simulink model "s0501_rollest_rideheight"  (R2021a)
settings: Solver=FixedStepAuto  StartTime=0.0  StopTime=10.0  FixedStep=0.001  RelTol=1e-3
libraries: CarMaker4SL x27, dspfdesign x1
settings Model: Creator=jason  LastModifiedBy=jason
settings ModelReferenceCC: ModelReferenceNumInstancesAllowed=Single

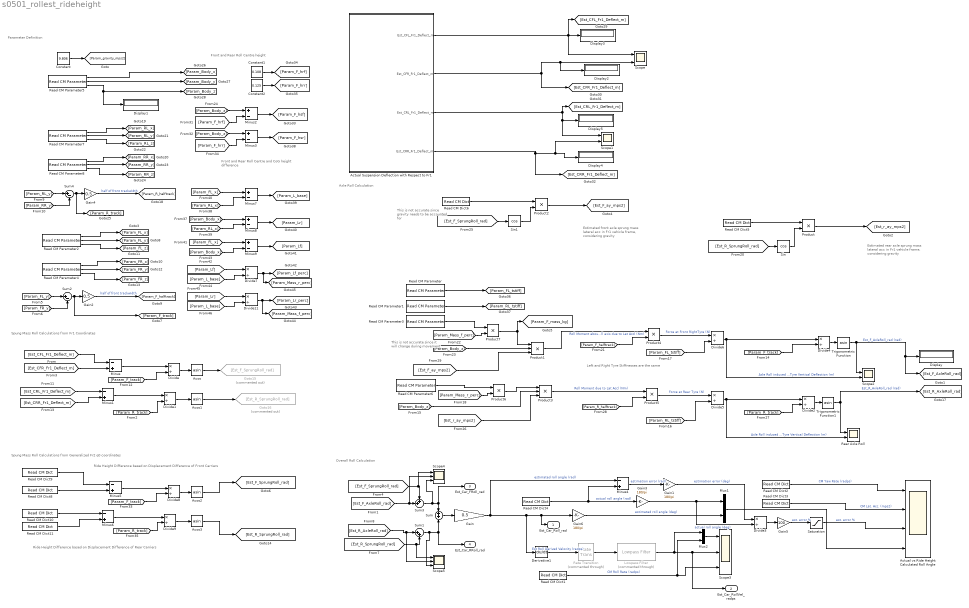
== system s0501_rollest_rideheight ==
  note: Ride Height Difference based on Displacement Difference of Rear Carriers
  note: Ride Height Difference based on Displacement Difference of Front Carriers
  note: Front and Rear Roll Centre height
  note: Overall Roll Calculation
  note: Parameter Definition
  note: Axle Roll Calculation
  note: Left and Right Tyre Stiffnesses are the same
  note: Spung Mass Roll Calculations from Fr1 Coordinates
  note: Estimated front axle sprung mass lateral acc in Fr1 vehicle frame, considering gravity
  note: Spung Mass Roll Calculations from Generalized Fr2 q0 coordinates
  note: This is not accurate since it will change during movement
  note: This is not accurate since gravity needs to be accounted for
  note: Estimated rear axle sprung mass lateral acc in Fr1 vehicle frame, considering gravity
  note: Front and Rear Roll Centre and CoG height difference
  Acos{,1..3} (4 alike) : Trigonometry  Operator=asin
  Actual Suspension Deflection with Respect to Fr1 : Subsystem
  Actual vs Ride Height Calculated Roll Angle : Scope  NumInputPorts=4
  Constant : Constant  Value=9.806
  Constant1 : Constant  Value=0.108
  Constant2 : Constant  Value=0.125
  Derivative1 : Derivative
  Display{,1..5} (6 alike) : Display
  Divide{,1..9,11} (11 alike) : Product  Inputs=*/
  Gain : Gain  Gain=0.5
  Gain1 : Gain  Gain=180/pi
      settings: AttributesFormatString=Gain = %<Gain>
  Gain2 : Gain  Gain=0.5
  Gain3 : Gain  Gain=180/pi
      settings: AttributesFormatString=Gain = %<Gain>
  Gain4 : Gain  Gain=0.5
  Gain5 : Gain  Gain=100
  Gain6 : Gain  Gain=180/pi
      settings: AttributesFormatString=Gain = %<Gain>
  Goto15 : Goto  Commented=on  GotoTag=Est_F_SprungRoll_rad
  Goto16 : Goto  Commented=on  GotoTag=Est_R_SprungRoll_rad
  Lowpass Filter : dspfdesign/Lowpass Filter  Commented=through  FilterType=FIR  DesignForMinimumOrder=on  FilterOrder=50  PassbandFrequency=1  StopbandFrequency=2000  PassbandRipple=0.1  StopbandAttenuation=180  InheritSampleRate=off  SampleRate=44100  SimulateUsing=Interpreted execution  roundingMode=Floor  coeffsDataTypeStr=fixdt(1,16)
  Minus{,1,4..6} (5 alike) : Sum  Inputs=-+
  Minus{2..3,7..9} (5 alike) : Sum  Inputs=+-
  Mux1 : Mux  Inputs=2
  Mux2 : Mux  Inputs=2
  Product{,2,4..7} (6 alike) : Product
  Product1 : Product  Inputs=3
  Product3 : Product  Inputs=3
  Rate Transition : RateTransition  Commented=through
  Read CM Dict1 : CarMaker4SL/Read CM Dict  xname=Car.RollVel  xsync=off  xstime=Continuous
  Read CM Dict10 : CarMaker4SL/Read CM Dict  xname=Car.CRL.q0  xsync=off  xstime=Continuous
  Read CM Dict11 : CarMaker4SL/Read CM Dict  xname=Car.CRR.q0  xsync=off  xstime=Continuous
  Read CM Dict2 : CarMaker4SL/Read CM Dict  xname=Car.YawRate  xsync=off  xstime=Continuous
  Read CM Dict3 : CarMaker4SL/Read CM Dict  xname=Car.ay  xsync=off  xstime=Continuous
  Read CM Dict4 : CarMaker4SL/Read CM Dict  xname=Car.Roll  xsync=off  xstime=Continuous
  Read CM Dict5 : CarMaker4SL/Read CM Dict  xname=Car.ay  xsync=off  xstime=Continuous
  Read CM Dict6 : CarMaker4SL/Read CM Dict  xname=Car.ay  xsync=off  xstime=Continuous
  Read CM Dict8 : CarMaker4SL/Read CM Dict  xname=Car.CFR.q0  xsync=off  xstime=Continuous
  Read CM Dict9 : CarMaker4SL/Read CM Dict  xname=Car.CFL.q0  xsync=off  xstime=Continuous
  Read CM Parameter : CarMaker4SL/Read CM Parameter  xfile=TireFL  xkey=Radial.Stiffness  xnout=1  xdefaults=0  xmuxed=on  xstime=Continuous
      settings: SourceProductName=CarMaker4SL
  Read CM Parameter1 : CarMaker4SL/Read CM Parameter  xfile=TireRL  xkey=Radial.Stiffness  xnout=1  xdefaults=0  xmuxed=on  xstime=Continuous
      settings: SourceProductName=CarMaker4SL
  Read CM Parameter2 : CarMaker4SL/Read CM Parameter  xfile=Vehicle  xkey=WheelCarrier.fl.pos  xnout=3  xdefaults=eps  xmuxed=off  xstime=Continuous
      settings: SourceProductName=CarMaker4SL
  Read CM Parameter3 : CarMaker4SL/Read CM Parameter  xfile=Vehicle  xkey=Body.mass  xnout=1  xdefaults=eps  xmuxed=off  xstime=Continuous
      settings: SourceProductName=CarMaker4SL
  Read CM Parameter4 : CarMaker4SL/Read CM Parameter  xfile=Vehicle  xkey=WheelCarrier.fr.pos  xnout=3  xdefaults=eps  xmuxed=off  xstime=Continuous
      settings: SourceProductName=CarMaker4SL
  Read CM Parameter5 : CarMaker4SL/Read CM Parameter  xfile=Vehicle  xkey=Body.pos  xnout=3  xdefaults=eps  xmuxed=off  xstime=Continuous
      settings: SourceProductName=CarMaker4SL
  Read CM Parameter6 : CarMaker4SL/Read CM Parameter  xfile=Vehicle  xkey=Body.mass  xnout=1  xdefaults=eps  xmuxed=off  xstime=Continuous
      settings: SourceProductName=CarMaker4SL
  Read CM Parameter7 : CarMaker4SL/Read CM Parameter  xfile=Vehicle  xkey=WheelCarrier.rl.pos  xnout=3  xdefaults=eps  xmuxed=off  xstime=Continuous
      settings: SourceProductName=CarMaker4SL
  Read CM Parameter8 : CarMaker4SL/Read CM Parameter  xfile=Vehicle  xkey=WheelCarrier.rr.pos  xnout=3  xdefaults=eps  xmuxed=off  xstime=Continuous
      settings: SourceProductName=CarMaker4SL
  Rear Axle Roll : Scope  NumInputPorts=2
  Saturation : Saturate  UpperLimit=100  LowerLimit=-100
  Scope{,3..5} (4 alike) : Scope  NumInputPorts=3
  Scope1 : Scope  NumInputPorts=2
  Scope2 : Scope  NumInputPorts=2
  Sin : Trigonometry  Operator=cos
  Sin1 : Trigonometry  Operator=cos
  Sum : Sum  Inputs=+|+
  Sum1 : Sum  Inputs=|++
  Sum2 : Sum  Inputs=|+-
  Sum3 : Sum  Inputs=++|
  Sum4 : Sum  Inputs=|+-
  Trigonometric Function : Trigonometry  Operator=asin
  Trigonometric Function1 : Trigonometry  Operator=asin
  Est_Car_Roll_rad : Outport
  Est_Car_RollVel_radps : Outport  Port=2
  Est_Car_FRoll_rad : Outport  Port=3
  Est_Car_RRoll_rad : Outport  Port=4
  wires:
  [Param_F_track] -> Divide8/2
  [Param_RR_y] -> Sum4/2
  Minus5/1 -> Divide8/1
  Read CM Dict3/1 -> Actual vs Ride Height Calculated Roll Angle/2  "CM Lat. Acc. (mps2)"
  Divide/1 -> Acos/1
  [Est_CRL_Fr1_Deflect_m] -> Minus1/1
  Rate Transition/1 -> Lowpass Filter/1
  Gain1/1 -> Divide3/1  "estimation error (deg)"
  Read CM Parameter3/1 -> Product7/1
  Sin/1 -> Product/2
  Read CM Dict2/1 -> Actual vs Ride Height Calculated Roll Angle/1  "CM Yaw Rate (radps)"
  Acos2/1 -> [Est_F_SprungRoll_rad]
  Acos3/1 -> [Est_R_SprungRoll_rad]
  [Est_F_SprungRoll_rad] -> Sin1/1
  Read CM Parameter4/2 -> [Param_FR_y]
  Gain/1 -> Minus4/1, Est_Car_Roll_rad/1, Gain6/1, Derivative1/1  "estimated roll angle (rad)"
  Divide9/1 -> Acos3/1
  Mux2/1 -> Scope3/1
  [Est_R_AxleRoll_rad] -> Scope5/2, Sum1/1
  [Est_r_ay_mps2] -> Product3/3
  Minus6/1 -> Divide9/1
  Actual Suspension Deflection with Respect to Fr1/1(Est_CFL_Fr1_Deflect_m) -> [Est_CFL_Fr1_Deflect_m], Scope/1, Display3/1
  Divide8/1 -> Acos2/1
  [Est_F_ay_mps2] -> Product1/3
  Acos/1 -> Goto15/1
  Read CM Dict10/1 -> Minus6/1
  Sin1/1 -> Product2/2
  Read CM Dict9/1 -> Minus5/1
  Read CM Dict8/1 -> Minus5/2
  Derivative1/1 -> Rate Transition/1  "Est Roll Derived Velocity (radps)"
  [Param_R_track] -> Divide9/2
  Mux1/1 -> Actual vs Ride Height Calculated Roll Angle/4
  Read CM Dict11/1 -> Minus6/2
  Read CM Dict1/1 -> Mux2/2, Scope3/3  "CM Roll Rate (radps)"
  [Param_F_track] -> Divide/2
  Trigonometric Function1/1 -> Rear Axle Roll/1, [Est_R_AxleRoll_rad]  "Est_R_AxleRoll_rad (rad)"
  [Est_CFL_Fr1_Deflect_m] -> Minus/1
  Read CM Parameter8/1 -> [Param_RR_x]
  Read CM Dict6/1 -> Product2/1
  Product/1 -> [Est_r_ay_mps2]
  Product3/1 -> Product5/1  "Roll Moment due to Lat Accl (Nm)"
  Product7/1 -> [Param_F_mass_kg], Product1/1
  Divide4/1 -> Trigonometric Function/1
  Product2/1 -> [Est_F_ay_mps2]
  Saturation/1 -> Actual vs Ride Height Calculated Roll Angle/3  "est. error %"
  [Est_CFR_Fr1_Deflect_m] -> Minus/2
  Actual Suspension Deflection with Respect to Fr1/4(Est_CRR_Fr1_Deflect_m) -> [Est_CRR_Fr1_Deflect_m], Display4/1, Scope1/2
  Read CM Parameter2/3 -> [Param_FL_z]
  Read CM Parameter/1 -> [Param_FL_tstiff]
  Gain2/1 -> [Param_F_halftrack]  "half of front trackwidth"
  Minus4/1 -> Gain1/1  "estimation error (rad)"
  Read CM Parameter2/1 -> [Param_FL_x]
  Sum3/1 -> Scope4/3, Est_Car_FRoll_rad/1, Sum/1
  [Param_FL_y] -> Sum2/1
  [Est_R_SprungRoll_rad] -> Sin/1
  Product6/1 -> Product3/1
  Constant/1 -> [Param_gravity_mps2]
  Product1/1 -> Product4/1  "Roll Moment about roll axis due to Lat Accl (Nm)"
  Sum4/1 -> Gain4/1, [Param_R_track]
  Acos1/1 -> Goto16/1
  Divide6/1 -> Divide4/1, Scope2/2  "Axle Roll induced Tyre Vertical Deflection (m)"
  Read CM Parameter1/1 -> [Param_RL_tstiff]
  Read CM Parameter6/1 -> Product6/1
  [Param_F_track] -> Divide4/2
  [Param_F_halftrack] -> Product4/2
  Product4/1 -> Divide6/1  "Force at Front RightTyre (N)"
  [Param_Body_z] -> Product3/2
  Product5/1 -> Divide5/1  "Force at Rear Tyre (N)"
  Divide2/1 -> Trigonometric Function1/1
  [Param_FL_tstiff] -> Divide6/2
  [Param_R_track] -> Divide2/2
  Trigonometric Function/1 -> Scope2/1, [Est_F_AxleRoll_rad], Display/1  "Est_F_AxleRoll_rad (rad)"
  Sum2/1 -> Gain2/1, [Param_F_track]
  Lowpass Filter/1 -> Mux2/1, Est_Car_RollVel_radps/1, Scope3/2
  Actual Suspension Deflection with Respect to Fr1/2(Est_CFR_Fr1_Deflect_m) -> Display2/1, Scope/3, [Est_CFR_Fr1_Deflect_m]
  Read CM Parameter5/2 -> [Param_Body_y]
  [Param_RL_tstiff] -> Divide5/2
  Divide3/1 -> Gain5/1
  [Param_Body_z] -> Product1/2
  [Est_CRR_Fr1_Deflect_m] -> Minus1/2
  Read CM Parameter5/1 -> [Param_Body_x]
  [Param_RL_y] -> Sum4/1
  Gain6/1 -> Mux1/2  "estimated roll angle (deg)"
  Divide5/1 -> Divide2/1, Rear Axle Roll/2  "Axle Roll induced Tyre Vertical Deflection (m)"
  Read CM Parameter2/2 -> [Param_FL_y]
  Read CM Parameter5/3 -> Display1/1, [Param_Body_z]
  [Est_R_SprungRoll_rad] -> Scope5/1, Sum1/2
  Minus1/1 -> Divide1/1
  Minus/1 -> Divide/1
  [Param_R_halftrack] -> Product5/2
  Gain4/1 -> [Param_R_halftrack]  "half of front trackwidth"
  [Param_FR_y] -> Sum2/2
  Gain3/1 -> Divide3/2, Mux1/1  "actual roll angle (deg)"
  Read CM Parameter8/2 -> [Param_RR_y]
  Read CM Parameter4/3 -> [Param_FR_z]
  Read CM Parameter4/1 -> [Param_FR_x]
  Sum1/1 -> Scope5/3, Est_Car_RRoll_rad/1, Sum/2
  Read CM Parameter7/1 -> [Param_RL_x]
  [Est_F_SprungRoll_rad] -> Scope4/1, Sum3/1
  Actual Suspension Deflection with Respect to Fr1/3(Est_CRL_Fr1_Deflect_m) -> [Est_CRL_Fr1_Deflect_m], Scope1/1, Display5/1
  Read CM Parameter8/3 -> [Param_RR_z]
  Read CM Parameter7/3 -> [Param_RL_z]
  [Param_R_track] -> Divide1/2
  [Est_F_AxleRoll_rad] -> Scope4/2, Sum3/2
  Read CM Dict4/1 -> Minus4/2, Gain3/1  "actual roll angle (rad)"
  Divide1/1 -> Acos1/1
  Sum/1 -> Gain/1
  Read CM Parameter7/2 -> [Param_RL_y]
  Read CM Dict5/1 -> Product/1
  Constant1/1 -> [Param_F_hrf]
  Constant2/1 -> [Param_F_hrr]
  [Param_F_hrf] -> Minus2/2
  [Param_Body_z] -> Minus2/1
  Minus2/1 -> [Param_F_hsf]
  Minus3/1 -> [Param_F_hsr]
  [Param_Body_z] -> Minus3/1
  [Param_F_hrr] -> Minus3/2
  [Param_Body_x] -> Minus8/1
  [Param_RL_x] -> Minus7/2
  [Param_FL_x] -> Minus7/1
  Minus7/1 -> [Param_L_base]
  [Param_RL_x] -> Minus8/2
  Minus8/1 -> [Param_Lr]
  [Param_FL_x] -> Minus9/1
  [Param_Body_x] -> Minus9/2
  Minus9/1 -> [Param_Lf]
  [Param_Lf] -> Divide7/1
  [Param_L_base] -> Divide7/2
  Divide7/1 -> [Param_Mass_r_perc], [Param_Lf_perc]
  Divide11/1 -> [Param_Mass_f_perc], [Param_Lr_perc]
  [Param_L_base] -> Divide11/2
  [Param_Lr] -> Divide11/1
  [Param_Mass_f_perc] -> Product7/2
  [Param_Mass_r_perc] -> Product6/2
  Gain5/1 -> Saturation/1  "est. error %"

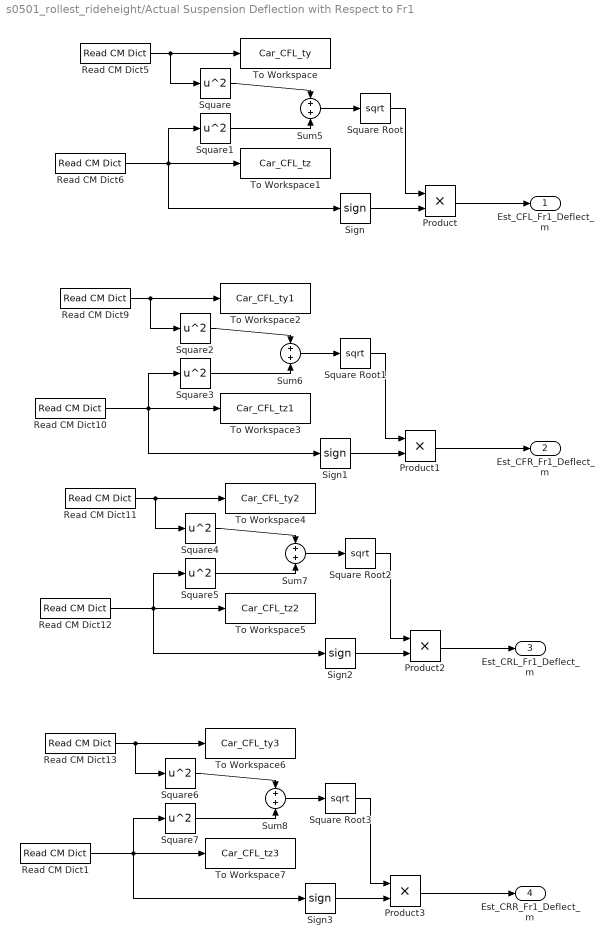
== system s0501_rollest_rideheight/Actual Suspension Deflection with Respect to Fr1 ==
  Product{,1..3} (4 alike) : Product
  Read CM Dict1 : CarMaker4SL/Read CM Dict  xname=Car.CRR.tz  xsync=off  xstime=Continuous
  Read CM Dict10 : CarMaker4SL/Read CM Dict  xname=Car.CFR.tz  xsync=off  xstime=Continuous
  Read CM Dict11 : CarMaker4SL/Read CM Dict  xname=Car.CRL.ty  xsync=off  xstime=Continuous
  Read CM Dict12 : CarMaker4SL/Read CM Dict  xname=Car.CRL.tz  xsync=off  xstime=Continuous
  Read CM Dict13 : CarMaker4SL/Read CM Dict  xname=Car.CRR.ty  xsync=off  xstime=Continuous
  Read CM Dict5 : CarMaker4SL/Read CM Dict  xname=Car.CFL.ty  xsync=off  xstime=Continuous
  Read CM Dict6 : CarMaker4SL/Read CM Dict  xname=Car.CFL.tz  xsync=off  xstime=Continuous
  Read CM Dict9 : CarMaker4SL/Read CM Dict  xname=Car.CFR.ty  xsync=off  xstime=Continuous
  Sign{,1..3} (4 alike) : Signum
  Square{,1..7} (8 alike) : Math  Operator=square  SaturateOnIntegerOverflow=on
  Square Root{,1..3} (4 alike) : Sqrt  SaturateOnIntegerOverflow=on
  Sum{5..8} (4 alike) : Sum
  To Workspace : ToWorkspace  VariableName=Car_CFL_ty  SampleTime=-1
  To Workspace1 : ToWorkspace  VariableName=Car_CFL_tz  SampleTime=-1
  To Workspace2 : ToWorkspace  VariableName=Car_CFL_ty1  SampleTime=-1
  To Workspace3 : ToWorkspace  VariableName=Car_CFL_tz1  SampleTime=-1
  To Workspace4 : ToWorkspace  VariableName=Car_CFL_ty2  SampleTime=-1
  To Workspace5 : ToWorkspace  VariableName=Car_CFL_tz2  SampleTime=-1
  To Workspace6 : ToWorkspace  VariableName=Car_CFL_ty3  SampleTime=-1
  To Workspace7 : ToWorkspace  VariableName=Car_CFL_tz3  SampleTime=-1
  Est_CFL_Fr1_Deflect_m : Outport
  Est_CFR_Fr1_Deflect_m : Outport  Port=2
  Est_CRL_Fr1_Deflect_m : Outport  Port=3
  Est_CRR_Fr1_Deflect_m : Outport  Port=4
  wires:
  Square Root2/1 -> Product2/1
  Square Root1/1 -> Product1/1
  Read CM Dict11/1 -> Square4/1, To Workspace4/1
  Square Root/1 -> Product/1
  Sign2/1 -> Product2/2
  Square/1 -> Sum5/1
  Sum5/1 -> Square Root/1
  Sign/1 -> Product/2
  Square5/1 -> Sum7/2
  Sum7/1 -> Square Root2/1
  Read CM Dict12/1 -> Sign2/1, Square5/1, To Workspace5/1
  Read CM Dict10/1 -> Sign1/1, Square3/1, To Workspace3/1
  Square1/1 -> Sum5/2
  Read CM Dict5/1 -> Square/1, To Workspace/1
  Read CM Dict6/1 -> Sign/1, Square1/1, To Workspace1/1
  Read CM Dict9/1 -> Square2/1, To Workspace2/1
  Square3/1 -> Sum6/2
  Sum8/1 -> Square Root3/1
  Read CM Dict13/1 -> Square6/1, To Workspace6/1
  Square4/1 -> Sum7/1
  Square2/1 -> Sum6/1
  Square6/1 -> Sum8/1
  Sum6/1 -> Square Root1/1
  Read CM Dict1/1 -> Sign3/1, Square7/1, To Workspace7/1
  Square Root3/1 -> Product3/1
  Product1/1 -> Est_CFR_Fr1_Deflect_m/1
  Sign3/1 -> Product3/2
  Sign1/1 -> Product1/2
  Square7/1 -> Sum8/2
  Product2/1 -> Est_CRL_Fr1_Deflect_m/1
  Product/1 -> Est_CFL_Fr1_Deflect_m/1
  Product3/1 -> Est_CRR_Fr1_Deflect_m/1
